simulink model "thuthapdulieu"  (Simulink 9.0)
settings: Solver=FixedStepAuto  StartTime=0.0  StopTime=10  FixedStep=0.1  RelTol=1e-3
undefined symbols (not defined in the file or in its folder): DiscIntNeverNeededParam, Kd, Ki, Kp
libraries: neural x73, simulink x1
(part 3 of 3)

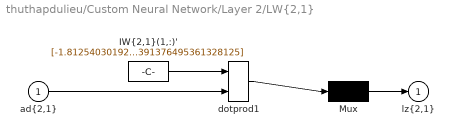
== system thuthapdulieu/Custom Neural Network/Layer 2/LW{2,1} ==
  "ad{2,1}" : Inport  PortDimensions=70  SampleTime=0.1
      mask Display: e = 0.06;c1 = [120 230 180]/255;c2 = ([120 230 180]+0)/(256+128);c3 = ([120 230 180]+128)/(256+128);patch([0 1 1 0],[0 0 1 1],c1);patch([0 1 1 1-e 1-e 0+e],[0 0 1 1-e 0+e 0+e],c2);patch([0 0 1 1-e 0+e 0+e],[0 1 1 1-e 1-e 0+e],c3);plot([0 1 1 0 0],[0 0 1 1 0]);
  "IW{2,1}(1,:)'" : Constant  Value=[-1.812540301928610819715004254248924553394317626953125;-0.783067774563714902313904531183652579784393310546875;1.7282546537496303873382430538185872137546539306640625;-1.768337850730142601918259970261715352535247802734375;-0.00084867761753041888288240368609649522113613784313201904296875;1.8145453772181399099139298414229415357112884521484375;1.808185838653518562324507001903839409351348876953125;0.325746624850705768228209535664063878357410430908203125;-1.3490229304267058463295825276873074471950531005859375;-1.4928014860368088445596868041320703923702239990234375;-0.5433017862464974978564669072511605918407440185546875;-2.542536697066942519285248636151663959026336669921875;0.682349555605218593967720153159461915493011474609375;-1.0212311607506734389971825294196605682373046875;-1.50976117165310075307615989004261791706085205078125;-0.428234337898064698624267521154251880943775177001953125;2.542089030992080278537059712107293307781219482421875;0.0661277009079081212750139684430905617773532867431640625;-1.4536382480736598221682243092800490558147430419921875;-1.4108388361791099896436207927763462066650390625;-2.69007651093312194490181354922242462635040283203125;2.11723297928103892928675122675485908985137939453125;-2.634946796891194598089214196079410612583160400390625;-2.6006578209713371307998386328108608722686767578125;-1.981972090746764170177129926742054522037506103515625;-2.288104555729395972463180441991426050662994384765625;-1.3741567334151441048817332557518966495990753173828125;2.0301092469432671094864417682401835918426513671875;0.5234385298199288882869950612075626850128173828125;-0.60959472254619562203714622228289954364299774169921875;0.2160861328700443007022613528533838689327239990234375;1.78298648158407413433224064647220075130462646484375;2.501724523979821146468793813255615532398223876953125;2.07202422075372982845919977989979088306427001953125;2.0783976209474008811639578198082745075225830078125;-2.10098574055938147608912913710810244083404541015625;-1.858874749897632572270822493010200560092926025390625;2.366128862938851273867157942731864750385284423828125;-2.57885675102125588864510064013302326202392578125;-0.63632445307096630049414898167015053331851959228515625;-0.73418194756482069163183723503607325255870819091796875;-0.1464121741155230693731681412828038446605205535888671875;0.5656991705413394466717136310762725770473480224609375;0.217109120317217019202615801987121812999248504638671875;-0.484681806529733971711237927593174390494823455810546875;-0.28006414862813377997241559569374658167362213134765625;1.3712997564679501039108799886889755725860595703125;-1.8788296143827272199899880433804355561733245849609375;0.2166594668105743803909746247882139869034290313720703125;-1.164179167988274254952330011292360723018646240234375;0.0327280017987356952602340243174694478511810302734375;-1.720709920198244535782805542112328112125396728515625;-1.48734801679905981330875874846242368221282958984375;2.740864035930460573808886692859232425689697265625;-0.5658109048947801422713155261590145528316497802734375;-0.86617591814750183321081067333579994738101959228515625;-1.598585569193331945569980234722606837749481201171875;-0.2085599974498757724905573240903322584927082061767578125;-0.565768288397226815078511208412237465381622314453125;-0.23020501751918531763152486746548675000667572021484375;-0.59685849009266489506586594870896078646183013916015625;2.370083604231890905822410786640830338001251220703125;-1.3088729217201748866727939457632601261138916015625;0.4339571332057452490715832027490250766277313232421875;-1.9927226819641978838859586176113225519657135009765625;-1.7279981566296302997187694927561096847057342529296875;-1.131995059172169248995487578213214874267578125;2.348898396347610884049572632648050785064697265625;1.40999057684707285176273217075504362583160400390625;3.1193836476378908884043994476087391376495361328125]
      mask Display: e = 0.06;c1 = [120 150 230]/255;c2 = ([120 150 230]+0)/383;c3 = ([120 150 230]+128)/383;patch([0 1 1 0],[0 0 1 1],c1);patch([0 1 1 1-e 1-e 0+e],[0 0 1 1-e 0+e 0+e],c2);patch([0 0 1 1-e 0+e 0+e],[0 1 1 1-e 1-e 0+e],c3);plot([0 1 1 0 0],[0 0 1 1 0]);disp('weights');
  Mux : Mux  Inputs=1
      mask Display: e = 0.06;c1 = [120 150 230]/255;c2 = ([120 150 230]+0)/383;c3 = ([120 150 230]+128)/383;patch([0 1 1 0],[0 0 1 1],c1);patch([0 1 1 1-e 1-e 0+e],[0 0 1 1-e 0+e 0+e],c2);patch([0 0 1 1-e 0+e 0+e],[0 1 1 1-e 1-e 0+e],c3);plot([0 1 1 0 0],[0 0 1 1 0]);disp('Mux');
  dotprod1 : neural/Weight Functions/dotprod
  "lz{2,1}" : Outport
      mask Display: e = 0.06;c1 = [120 230 180]/255;c2 = ([120 230 180]+0)/(256+128);c3 = ([120 230 180]+128)/(256+128);patch([0 1 1 0],[0 0 1 1],c1);patch([0 1 1 1-e 1-e 0+e],[0 0 1 1-e 0+e 0+e],c2);patch([0 0 1 1-e 0+e 0+e],[0 1 1 1-e 1-e 0+e],c3);plot([0 1 1 0 0],[0 0 1 1 0]);
  wires:
  "IW{2,1}(1,:)'"/1 -> dotprod1/1
  "ad{2,1}"/1 -> dotprod1/2
  dotprod1/1 -> Mux/1
  Mux/1 -> "lz{2,1}"/1
